simulink subsystem "controller"  (R2020a)
settings: Solver=VariableStepAuto  StartTime=0.0  StopTime=10.0  RelTol=1e-3
values from neighbouring files (symbols this model uses):
  Eqlut = zeros(slotsAngle, slotsSpeed, 2)    [LUTScript.m]    (also in Lutscript.m = zeros(10,13,2); generateLUTs.m)
  Klut = zeros(slotsAngle, slotsSpeed, 2)    [LUTScript.m]    (also in Lutscript.m = zeros(10,13,2); generateLUTs.m)
settings Model: Creator=Fil  LastModifiedBy=filip

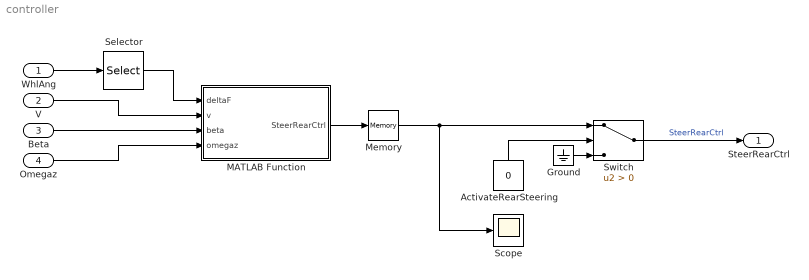
== system controller ==
  WhlAng : Inport
  V : Inport  Port=2
  Beta : Inport  Port=3
  Omegaz : Inport  Port=4
  ActivateRearSteering : Constant  Value=0
  Ground : Ground
  MATLAB Function : MATLAB Function  TreatAsAtomicUnit=on
      settings: MinAlgLoopOccurrences=on
  Memory : Memory
  Scope : Scope
  Selector : Selector  InputPortWidth=4  IndexOptions=Index vector (dialog)  Indices=[1 2]  OutputSizes=1
  Switch : Switch  Criteria=u2 > Threshold
  SteerRearCtrl : Outport
  wires:
  MATLAB Function/1(SteerRearCtrl) -> Memory/1
  WhlAng/1 -> Selector/1
  Memory/1 -> Scope/1, Switch/1
  Beta/1 -> MATLAB Function/3(beta)
  Omegaz/1 -> MATLAB Function/4(omegaz)
  Selector/1 -> MATLAB Function/1(deltaF)
  V/1 -> MATLAB Function/2(v)
  ActivateRearSteering/1 -> Switch/2
  Switch/1 -> SteerRearCtrl/1  "SteerRearCtrl"
  Ground/1 -> Switch/3

== matlab function controller/MATLAB Function ==
  data: deltaF input; SteerRearCtrl output; v input; beta input; omegaz input; Klut parameter; Eqlut parameter
function SteerRearCtrl = optRear(deltaF,v,beta,omegaz, Klut, Eqlut)
K = zeros(2);
Ref = zeros(2);

% Select LUT indexes
i = (round(deltaF/3));
j = round(v/10);

% Extract form LUTs
K = Klut(i+1,j+1,:);
Ref = Eqlut(i+1,j+1,:);

% Equilibrium references from LUT
betaeq = Ref(1)
omegazeq = Ref(2)

SteerRearCtrl =  (K(1)*(beta-betaeq)) + (K(2)*(omegaz-omegazeq));
